simulink model "Copy_of_two_phase_main_loop"  (R2025b)
settings: Solver=VariableStepAuto  StartTime=0.0  StopTime=4000
undefined symbols (not defined in the file): cfg, u_cmd
libraries: nesl_utility x21, fl_lib x20, SimscapeFluids_lib x7, slpidlib x1
settings Model: LastModifiedBy=altoa
settings OptimizationCC: ZeroExternalMemoryAtStartup=off  ZeroInternalMemoryAtStartup=off
settings RTWCC: GenerateReport=on  LaunchReport=on  TargetLang=C++  CheckMdlBeforeBuild=Error
settings GRTTargetCC: TargetLangStandard=C++11 (ISO)  CodeInterfacePackaging=C++ class  SubcomponentCodeInterfacePackaging=C++ class

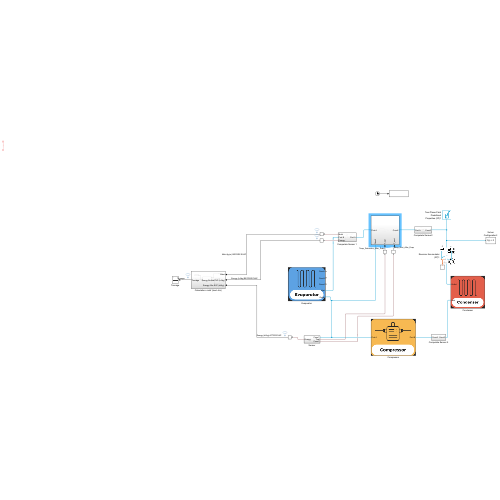
[thumbnail: Simulink's stored preview of the top-level diagram]
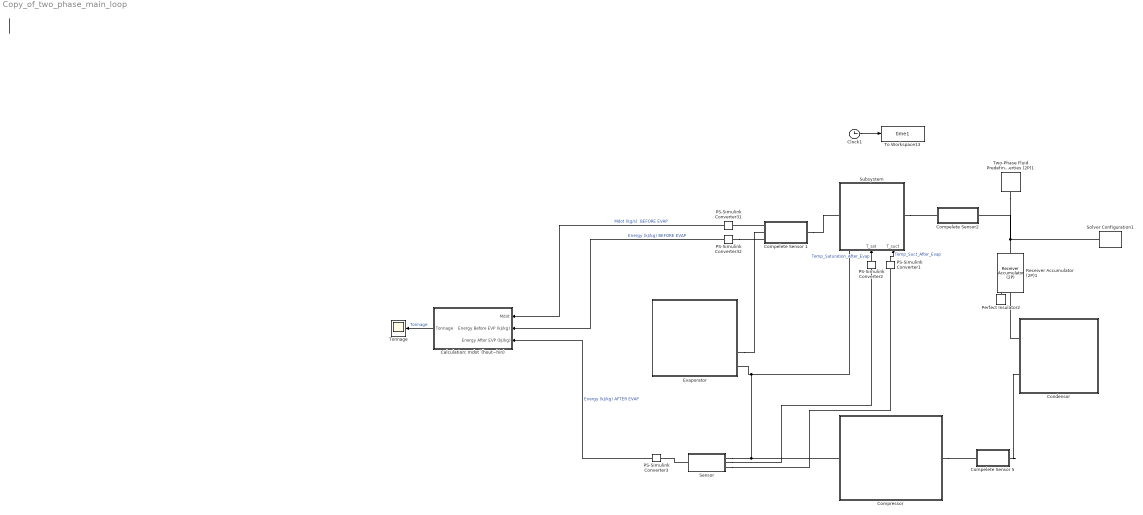
== system Copy_of_two_phase_main_loop ==
  Calculation: mdot˙(hout​−hin​) : Subsystem
  Clock1 : Clock
  Compelete Sensor 1 : Subsystem
  Compelete Sensor 5 : Subsystem
  Compelete Sensor2 : Subsystem
  Compressor : Subsystem
      mask Display: image('models\Icon\Compressor.png');
  Condensor : Subsystem
      mask Display: image('models\Icon\Condenser.png');
  Evaporator : Subsystem
      mask Display: image("models\Icon\Evaporator.png");
  PS-Simulink Converter{1..3,31..32} (5 alike) : nesl_utility/PS-Simulink Converter  PhysicalDomain=network_engine_domain  SubClassName=ps_output  LeftPortType=input  RightPortType=output  PseudoPeriodic=off  Frequencies=[]  VectorFormat=inherit  Unit=inherit  AffineConversion=off
  Perfect Insulator2 : fl_lib/Thermal/Thermal Elements/Perfect Insulator  T_specify=off  T_priority=None  T=293.15 K  T_nominal_specify=off  T_nominal_value=1  T_nominal_unit=K
  Receiver Accumulator (2P)1 : SimscapeFluids_lib/Two-Phase Fluid/Tanks & Accumulators/Receiver Accumulator (2P)  volume=pi*0.15^2/4 * 0.5 m^3  tank_area=pi*0.15^2/4 m^2  area_AV=pi*0.02^2/4 m^2  area_BV=pi*0.02^2/4 m^2  area_AL=pi*0.02^2/4 m^2  area_BL=pi*0.02^2/4 m^2  V_frac_liq_error=simscape.enum.assert.action.none  V_frac_liq_min=0.05  V_frac_liq_max=0.95  V_frac_smooth=0.05  p_crit_error=simscape.enum.assert.action.error  hc_vap=20 W/(K*m^2)  hc_liq=100 W/(K*m^2)  p_init=2.734 MPa  fraction_spec=fluids.two_phase_fluid.tanks_accumulators.enum.LiquidFractionSpec.Volume  M_frac_liq_init=0.5  V_frac_liq_init=0.5  saturated_init=true  energy_spec=fluids.two_phase_fluid.tanks_accumulators.enum.EnergySpec.SubcoolingSuperheating  delta_T_sub_init=5 deltaK  delta_T_sup_init=5 deltaK  T_liq_init=368.15 K  T_vap_init=378.15 K  h_liq_init=400 kJ/kg  h_vap_init=2700 kJ/kg  u_liq_init=400 kJ/kg  u_vap_init=2700 kJ/kg  tau_vap_cond=1 s
      settings: InternalSimscapePortConfiguration="{\"Bottom\":[],\"Left\":[{\"id\":\"AV\",\"label\":\"AV\",\"type\":\"foundation.two_phase_fluid.two_phase_fluid\"},{\"id\":\"AL\",\"label\":\"AL\",\"type\":\"foundation.two_phase_fluid.two_phase_fluid\"},{\"id\":\"H\",\"label\":\"H\",\"type\":\"foundation.thermal.thermal\"}],\"Right\":[{\"id\":\"BV\",\"label\":\"BV\",\"type\":\"foundation.two_phase_fluid.two_phase_fluid\"},{\"id\":\"BL\",\"label\":\"BL\",\"type\":\"foundation.two_phase_fluid.two_phase_fluid\"},{\"id\":\"L\",\"label\":\"L\",\"type\":\"output\"}],\"Top\":[]}"
  Sensor : Subsystem
  Solver Configuration1 : nesl_utility/Solver Configuration  PhysicalDomain=network_engine_domain  SubClassName=solver  LeftPortType=input  RightPortType=generic  Tones=[]  Harmonics=[]  SimulateNoise=off  Profile=off  UseLocalSampling=off  EnableSwitchedLinearOptims=on  FrequencyDomain=off  UseCCode=off  RelTol=0.001  AbsTol=0.001  MinStep=1e-09  ToWorkspace=off  RevertToSquareIcSolve=off  NumHomotopyIterations=100  PhasorMode=off  PhasorModeNumHarmonics=1  ConsistencySolver=NEWTON_FTOL  IndexReductionMethod=DerivativeReplacement  DoDC=off  ResidualTolerance=1e-09  ConsistencyTolSource=GLOBAL  ConsistencyAbsTol=0.001  ConsistencyRelTol=0.001  ConsistencyTolFactor=0.001  UseLocalSolver=off  LocalSolverChoice=NE_BACKWARD_EULER_ADVANCER  ResolveIndetEquations=on  FunctionEvalNumThread=1  LocalSolverSampleTime=0.001  DoFixedCost=off  MaxNonlinIter=3  MaxModeIter=2  ComputeImpulses=off  ImpulseIterations=2  LinearAlgebra=auto  LinearAlgebraNumThread=0  EquationFormulation=NE_TIME_EF  DelaysMemoryBudget=1024  AutomaticFiltering=on  FilteringTimeConstant=0.001  PartitionStorageMethod=AS_NEEDED  PartitionMemoryBudget=1024  PartitionMethod=ROBUST  MultibodyUseLocalSolver=off  MultibodyLocalSolverChoice=ODE1  MultibodyLocalSolverSampleTime=0.001
  Subsystem : Subsystem
      settings: PortSchema="{\"entries\":[{\"content\":{\"sides\":[{\"content\":{\"connectorIds\":[\"LConn1\"]},\"type\":\"ConnectorPlacement.EquallySpacedRectSide\",\"uuid\":\"f5d6d53e-9d0c-4e0a-9987-2cecb9078f40\"},{\"content\":{\"connectorIds\":[\"RConn1\"],\"side\":\"RIGHT\"},\"type\":\"ConnectorPlacement.EquallySpacedRectSide\",\"uuid\":\"a442d892-4933-408d-9a01-d57d967d5942\"},{\"content\":{\"side\":\"TOP\"},\"type\":\"ConnectorPlacement.EquallySpacedRectSide\",\"uuid\":\"9d728b22-2b02-46e5-9d77-02223002d615\"},{\"content\":{\"connectorIds\":[\"In1\",\"In2\",\"RConn2\"],\"side\":\"BOTTOM\"},\"type\":\"ConnectorPlacement.EquallySpacedRectSide\",\"uuid\":\"bdbf34ec-8662-4590-a2f3-7ce9740bfea5\"}]},\"type\":\"ConnectorPlacement.EquallySpacedConnector\",\"uuid\":\"3394dac1-307d-4ba8-b50d-5218a2108d88\"}],\"packageUris\":[\"http://schema.mathworks.com/mf0/Connector/R2020b\"],\"version\":\"1.0\"}"
  To Workspace13 : ToWorkspace  VariableName=time1  SampleTime=-1
  Tonnage : Scope
      settings: ActiveDisplayYMinimum=2.6000959343820402  ActiveDisplayYMaximum=3.4572001399689993  DataLoggingVariableName=ScopeData29
  Two-Phase Fluid Predefined Properties (2P)1 : SimscapeFluids_lib/Two-Phase Fluid/Utilities/Two-Phase Fluid Predefined Properties (2P)  fluid=fluids.two_phase_fluid.utilities.enum.Fluid.R32  p_atm=0.101325 MPa  properties_range_check=simscape.enum.assert.action.error  q_rev=0.01 Pa
  wires:
  Clock1/1 -> To Workspace13/1
  PS-Simulink Converter32/1 -> Calculation: mdot˙(hout​−hin​)/2(Energy Before EVP (kJ/kg))  "Energy (kJ/kg) BEFORE EVAP"
  Calculation: mdot˙(hout​−hin​)/1(Tonnage) -> Tonnage/1  "Tonnage"
  PS-Simulink Converter31/1 -> Calculation: mdot˙(hout​−hin​)/1(Mdot)  "Mdot (kg/s)  BEFORE EVAP"
  PS-Simulink Converter3/1 -> Calculation: mdot˙(hout​−hin​)/3("Energy After EVP (kJ/kg) ")  "Energy (kJ/kg) AFTER EVAP"
  PS-Simulink Converter1/1 -> Subsystem/1(T_suct)  "Temp_Suct_After_Evap"
  PS-Simulink Converter2/1 -> Subsystem/2(T_sat)  "Temp_Saturation_After_Evap"
  connections:
  ?
  Receiver Accumulator (2P)1/RConn2 -- Two-Phase Fluid Predefined Properties (2P)1/RConn1 -- Compelete Sensor2/LConn1 -- Solver Configuration1/RConn1
  Compelete Sensor 5/RConn1 -- Condensor/LConn2
  Perfect Insulator2/LConn1 -- Receiver Accumulator (2P)1/LConn3
  Compelete Sensor 1/RConn1 -- PS-Simulink Converter31/LConn1
  Evaporator/LConn4 -- Compelete Sensor 1/RConn2
  PS-Simulink Converter32/LConn1 -- Compelete Sensor 1/RConn3
  Condensor/LConn1 -- Receiver Accumulator (2P)1/LConn2
  Compressor/RConn1 -- Compelete Sensor 5/LConn1
  Sensor/RConn1 -- PS-Simulink Converter3/LConn1
  Sensor/LConn2 -- PS-Simulink Converter2/LConn1
  Sensor/LConn3 -- PS-Simulink Converter1/LConn1
  Sensor/LConn1 -- Evaporator/LConn5 -- Subsystem/RConn2 -- Compressor/LConn1
  Compelete Sensor 1/LConn1 -- Subsystem/RConn1
  Subsystem/LConn1 -- Compelete Sensor2/RConn1

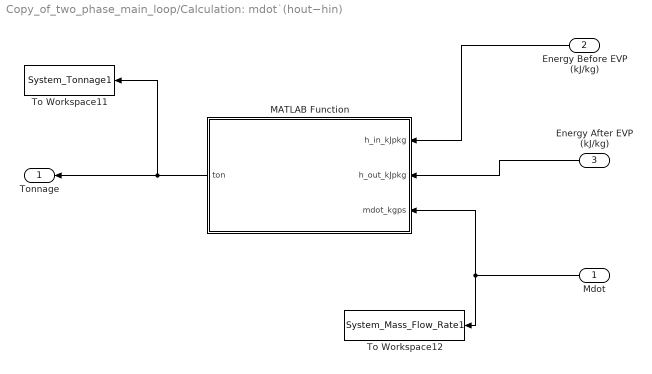
== system Copy_of_two_phase_main_loop/Calculation: mdot˙(hout​−hin​) ==
  Mdot : Inport
  Energy Before EVP (kJ/kg) : Inport  Port=2
  "Energy After EVP (kJ/kg) " : Inport  Port=3
  MATLAB Function : MATLAB Function  TreatAsAtomicUnit=on
  To Workspace11 : ToWorkspace  VariableName=System_Tonnage1  SampleTime=-1
  To Workspace12 : ToWorkspace  VariableName=System_Mass_Flow_Rate1  SampleTime=-1
  Tonnage : Outport
  wires:
  MATLAB Function/1(ton) -> To Workspace11/1, Tonnage/1
  Mdot/1 -> To Workspace12/1, MATLAB Function/3(mdot_kgps)
  Energy Before EVP (kJ/kg)/1 -> MATLAB Function/1(h_in_kJpkg)
  "Energy After EVP (kJ/kg) "/1 -> MATLAB Function/2(h_out_kJpkg)

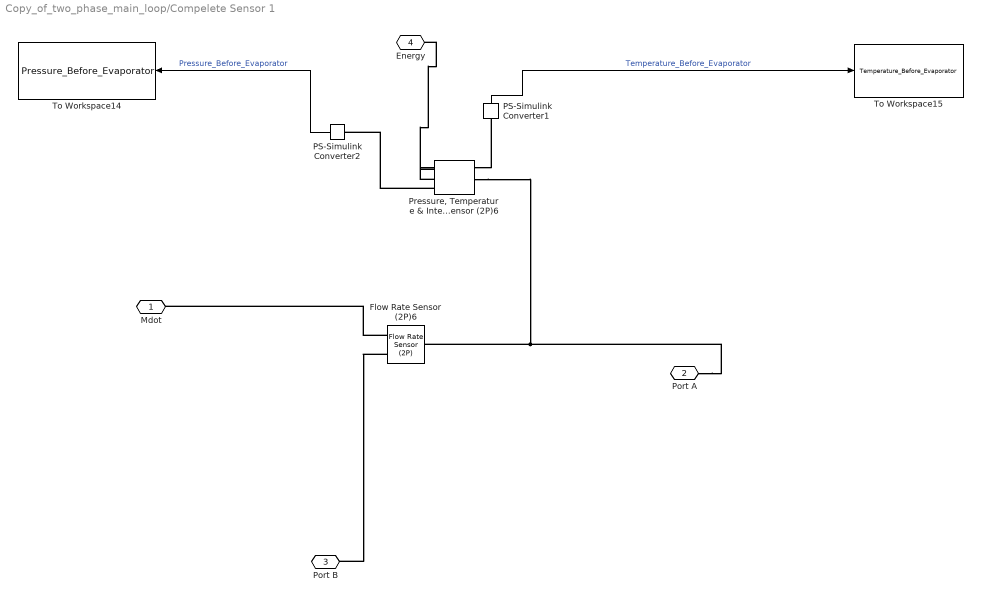
== system Copy_of_two_phase_main_loop/Compelete Sensor 1 ==
  Flow Rate Sensor (2P)6 : fl_lib/Two-Phase Fluid/Sensors/Flow Rate Sensor (2P)  mass_flow_measure=true  volumetric_flow_measure=false  energy_flow_measure=false
      settings: InternalSimscapePortConfiguration="{\"Bottom\":[],\"Left\":[{\"id\":\"A\",\"label\":\"A\",\"type\":\"foundation.two_phase_fluid.two_phase_fluid\"}],\"Right\":[{\"id\":\"B\",\"label\":\"B\",\"type\":\"foundation.two_phase_fluid.two_phase_fluid\"},{\"id\":\"M\",\"label\":\"M\",\"type\":\"output\"}],\"Top\":[]}"
  PS-Simulink Converter1 : nesl_utility/PS-Simulink Converter  PhysicalDomain=network_engine_domain  SubClassName=ps_output  LeftPortType=input  RightPortType=output  PseudoPeriodic=off  Frequencies=[]  VectorFormat=inherit  Unit=inherit  AffineConversion=off
  PS-Simulink Converter2 : nesl_utility/PS-Simulink Converter  PhysicalDomain=network_engine_domain  SubClassName=ps_output  LeftPortType=input  RightPortType=output  PseudoPeriodic=off  Frequencies=[]  VectorFormat=inherit  Unit=inherit  AffineConversion=off
  "Pressure, Temperature & Internal Energy Sensor (2P)6" : fl_lib/Two-Phase Fluid/Sensors/Pressure, Temperature & Internal Energy Sensor (2P)  reference=foundation.enum.MeasurementReference.absolute  pressure=true  pressure_spec=foundation.enum.PressureMeasementSpec.Absolute  temperature=true  internal_energy=true
      settings: InternalSimscapePortConfiguration="{\"Bottom\":[{\"id\":\"T\",\"label\":\"T\",\"type\":\"output\"},{\"id\":\"U\",\"label\":\"U\",\"type\":\"output\"}],\"Left\":[{\"id\":\"A\",\"label\":\"A\",\"type\":\"foundation.two_phase_fluid.two_phase_fluid\"}],\"Right\":[{\"id\":\"Pa\",\"label\":\"Pa\",\"type\":\"output\"}],\"Top\":[]}"
  To Workspace14 : ToWorkspace  VariableName=Pressure_Before_Evaporator  SampleTime=-1
  To Workspace15 : ToWorkspace  VariableName=Temperature_Before_Evaporator  SampleTime=-1
  Mdot : PMIOPort  Side=Right
  Port A : PMIOPort  Port=2  Side=Left
  Port B : PMIOPort  Port=3  Side=Right
  "Energy " : PMIOPort  Port=4  Side=Right
  wires:
  PS-Simulink Converter1/1 -> To Workspace15/1  "Temperature_Before_Evaporator"
  PS-Simulink Converter2/1 -> To Workspace14/1  "Pressure_Before_Evaporator"
  connections:
  Port A/RConn1 -- "Pressure, Temperature & Internal Energy Sensor (2P)6"/LConn1 -- Flow Rate Sensor (2P)6/LConn1
  Flow Rate Sensor (2P)6/RConn1 -- Port B/RConn1
  Flow Rate Sensor (2P)6/RConn2 -- Mdot/RConn1
  "Pressure, Temperature & Internal Energy Sensor (2P)6"/RConn3 -- "Energy "/RConn1
  "Pressure, Temperature & Internal Energy Sensor (2P)6"/RConn2 -- PS-Simulink Converter1/LConn1
  "Pressure, Temperature & Internal Energy Sensor (2P)6"/RConn1 -- PS-Simulink Converter2/LConn1

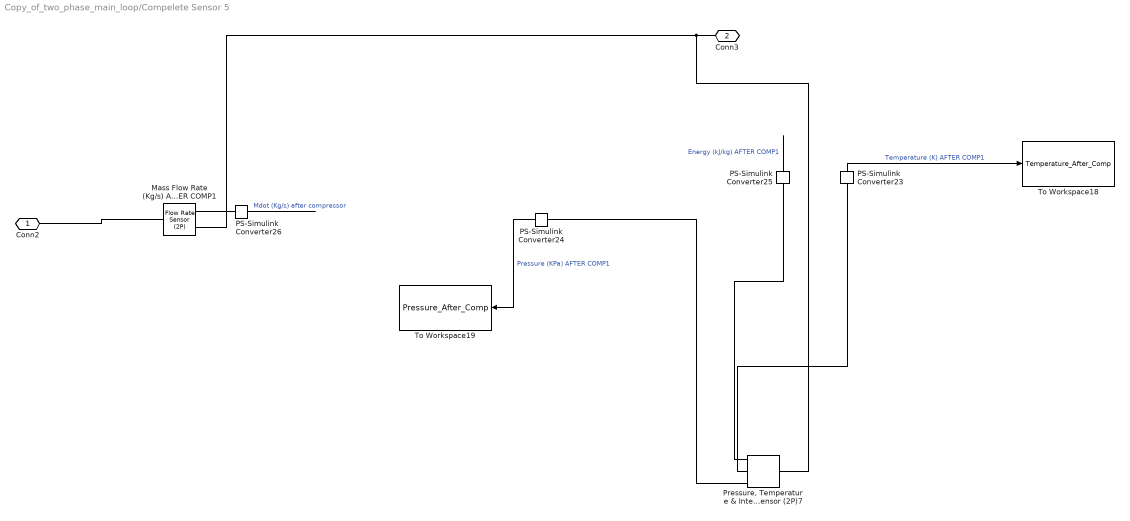
== system Copy_of_two_phase_main_loop/Compelete Sensor 5 ==
  Mass Flow Rate (Kg/s) AFTER COMP1 : fl_lib/Two-Phase Fluid/Sensors/Flow Rate Sensor (2P)  mass_flow_measure=true  volumetric_flow_measure=false  energy_flow_measure=false
      settings: InternalSimscapePortConfiguration="{\"Bottom\":[],\"Left\":[{\"id\":\"A\",\"label\":\"A\",\"type\":\"foundation.two_phase_fluid.two_phase_fluid\"}],\"Right\":[{\"id\":\"B\",\"label\":\"B\",\"type\":\"foundation.two_phase_fluid.two_phase_fluid\"},{\"id\":\"M\",\"label\":\"M\",\"type\":\"output\"}],\"Top\":[]}"
  PS-Simulink Converter{23..26} (4 alike) : nesl_utility/PS-Simulink Converter  PhysicalDomain=network_engine_domain  SubClassName=ps_output  LeftPortType=input  RightPortType=output  PseudoPeriodic=off  Frequencies=[]  VectorFormat=inherit  Unit=inherit  AffineConversion=off
  "Pressure, Temperature & Internal Energy Sensor (2P)7" : fl_lib/Two-Phase Fluid/Sensors/Pressure, Temperature & Internal Energy Sensor (2P)  reference=foundation.enum.MeasurementReference.absolute  pressure=true  pressure_spec=foundation.enum.PressureMeasementSpec.Absolute  temperature=true  internal_energy=true
      settings: InternalSimscapePortConfiguration="{\"Bottom\":[{\"id\":\"T\",\"label\":\"T\",\"type\":\"output\"},{\"id\":\"U\",\"label\":\"U\",\"type\":\"output\"}],\"Left\":[{\"id\":\"A\",\"label\":\"A\",\"type\":\"foundation.two_phase_fluid.two_phase_fluid\"}],\"Right\":[{\"id\":\"Pa\",\"label\":\"Pa\",\"type\":\"output\"}],\"Top\":[]}"
  To Workspace18 : ToWorkspace  VariableName=Temperature_After_Comp  SampleTime=-1
  To Workspace19 : ToWorkspace  VariableName=Pressure_After_Comp  SampleTime=-1
  Conn2 : PMIOPort  Side=Left
  Conn3 : PMIOPort  Port=2  Side=Right
  wires:
  PS-Simulink Converter26/1 -> ?  "Mdot (Kg/s) after compressor"
  PS-Simulink Converter24/1 -> To Workspace19/1  "Pressure (KPa) AFTER COMP1"
  PS-Simulink Converter23/1 -> To Workspace18/1  "Temperature (K) AFTER COMP1"
  PS-Simulink Converter25/1 -> ?  "Energy (kJ/kg) AFTER COMP1"
  connections:
  Conn2/RConn1 -- Mass Flow Rate (Kg/s) AFTER COMP1/LConn1
  PS-Simulink Converter26/LConn1 -- Mass Flow Rate (Kg/s) AFTER COMP1/RConn2
  Mass Flow Rate (Kg/s) AFTER COMP1/RConn1 -- Conn3/RConn1 -- "Pressure, Temperature & Internal Energy Sensor (2P)7"/LConn1
  PS-Simulink Converter23/LConn1 -- "Pressure, Temperature & Internal Energy Sensor (2P)7"/RConn2
  PS-Simulink Converter25/LConn1 -- "Pressure, Temperature & Internal Energy Sensor (2P)7"/RConn3
  PS-Simulink Converter24/LConn1 -- "Pressure, Temperature & Internal Energy Sensor (2P)7"/RConn1

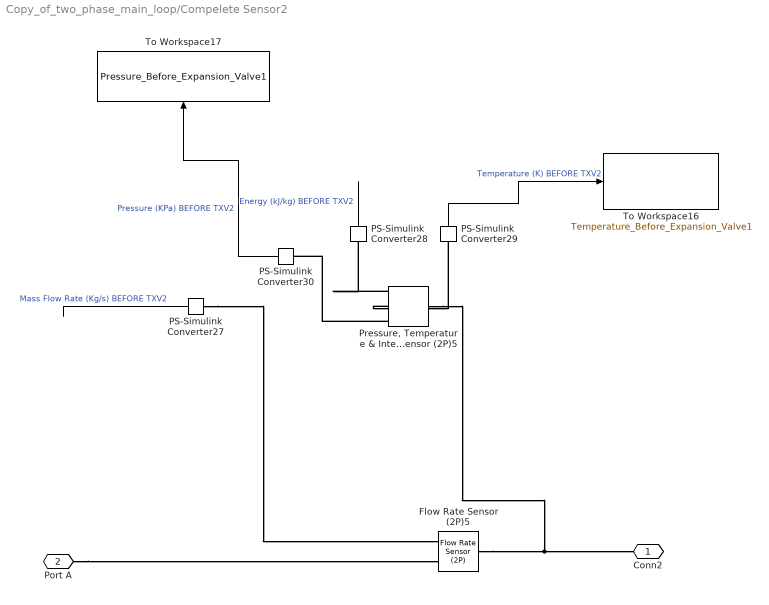
== system Copy_of_two_phase_main_loop/Compelete Sensor2 ==
  Flow Rate Sensor (2P)5 : fl_lib/Two-Phase Fluid/Sensors/Flow Rate Sensor (2P)  mass_flow_measure=true  volumetric_flow_measure=false  energy_flow_measure=false
      settings: InternalSimscapePortConfiguration="{\"Bottom\":[],\"Left\":[{\"id\":\"A\",\"label\":\"A\",\"type\":\"foundation.two_phase_fluid.two_phase_fluid\"}],\"Right\":[{\"id\":\"B\",\"label\":\"B\",\"type\":\"foundation.two_phase_fluid.two_phase_fluid\"},{\"id\":\"M\",\"label\":\"M\",\"type\":\"output\"}],\"Top\":[]}"
  PS-Simulink Converter{27..30} (4 alike) : nesl_utility/PS-Simulink Converter  PhysicalDomain=network_engine_domain  SubClassName=ps_output  LeftPortType=input  RightPortType=output  PseudoPeriodic=off  Frequencies=[]  VectorFormat=inherit  Unit=inherit  AffineConversion=off
  "Pressure, Temperature & Internal Energy Sensor (2P)5" : fl_lib/Two-Phase Fluid/Sensors/Pressure, Temperature & Internal Energy Sensor (2P)  reference=foundation.enum.MeasurementReference.absolute  pressure=true  pressure_spec=foundation.enum.PressureMeasementSpec.Absolute  temperature=true  internal_energy=true
      settings: InternalSimscapePortConfiguration="{\"Bottom\":[{\"id\":\"T\",\"label\":\"T\",\"type\":\"output\"},{\"id\":\"U\",\"label\":\"U\",\"type\":\"output\"}],\"Left\":[{\"id\":\"A\",\"label\":\"A\",\"type\":\"foundation.two_phase_fluid.two_phase_fluid\"}],\"Right\":[{\"id\":\"Pa\",\"label\":\"Pa\",\"type\":\"output\"}],\"Top\":[]}"
  To Workspace16 : ToWorkspace  VariableName=Temperature_Before_Expansion_Valve1  SampleTime=-1
  To Workspace17 : ToWorkspace  VariableName=Pressure_Before_Expansion_Valve1  SampleTime=-1
  Conn2 : PMIOPort  Side=Left
  Port A : PMIOPort  Port=2  Side=Right
  wires:
  PS-Simulink Converter30/1 -> To Workspace17/1  "Pressure (KPa) BEFORE TXV2"
  PS-Simulink Converter29/1 -> To Workspace16/1  "Temperature (K) BEFORE TXV2"
  PS-Simulink Converter27/1 -> ?  "Mass Flow Rate (Kg/s) BEFORE TXV2"
  PS-Simulink Converter28/1 -> ?  "Energy (kJ/kg) BEFORE TXV2"
  connections:
  Port A/RConn1 -- Flow Rate Sensor (2P)5/RConn1
  PS-Simulink Converter27/LConn1 -- Flow Rate Sensor (2P)5/RConn2
  Flow Rate Sensor (2P)5/LConn1 -- "Pressure, Temperature & Internal Energy Sensor (2P)5"/LConn1 -- Conn2/RConn1
  "Pressure, Temperature & Internal Energy Sensor (2P)5"/RConn1 -- PS-Simulink Converter30/LConn1
  "Pressure, Temperature & Internal Energy Sensor (2P)5"/RConn2 -- PS-Simulink Converter29/LConn1
  "Pressure, Temperature & Internal Energy Sensor (2P)5"/RConn3 -- PS-Simulink Converter28/LConn1

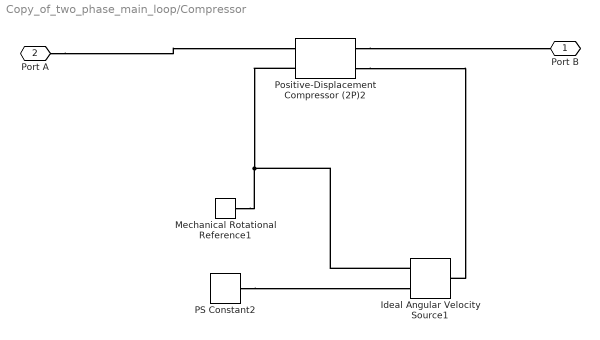
== system Copy_of_two_phase_main_loop/Compressor ==
  Ideal Angular Velocity Source1 : fl_lib/Mechanical/Mechanical Sources/Ideal Angular Velocity Source
  Mechanical Rotational Reference1 : fl_lib/Mechanical/Rotational Elements/Mechanical Rotational Reference
  PS Constant2 : fl_lib/Physical Signals/Sources/PS Constant  constant=220 Hz
  Positive-Displacement Compressor (2P)2 : SimscapeFluids_lib/Two-Phase Fluid/Fluid Machines/Positive-Displacement Compressor (2P)  dispSpec=fluids.two_phase_fluid.fluid_machines.enum.DisplacementSpecification.FlowSpeed  v_disp=130 cm^3/rev  mdot_nom=0.013 kg/s  omega_nom=60 Hz  efficiencySpec=fluids.two_phase_fluid.fluid_machines.enum.VolumetricEfficiencyParameterization.Analytical  thermodynamicModelSpec=fluids.two_phase_fluid.fluid_machines.enum.ThermodynamicModel.Polytropic  n=1.2  eta_isen=0.65  eta_isen_TLU=[.95, .9, .85, .8, .75; .925, .875, .825, .775, .725; .875, .825, .775, .725, .675; .75, .7, .65, .6, .55]  eta_vol_nom=0.9  pr_TLU=[2, 4, 6, 8]  omega_TLU=[800, 1500, 2800, 3300, 4000] rpm  eta_vol_TLU=[.95, .9, .85, .8, .75; .925, .875, .825, .775, .725; .875, .825, .775, .725, .675; .75, .7, .65, .6, .55]  nominalSpec=fluids.two_phase_fluid.fluid_machines.enum.NominalConditionsSpecification.SaturationTemperatures  pr_nom=5  p_in_nom=0.101325 MPa  T_in_nom=373.15 K  T_evap_nom=5 degC  T_cond_nom=45 degC  delta_T_nom=5 deltaK  mechanical_efficiency=0.9  area_A=pi*0.02^2/4 m^2  area_B=pi*0.02^2/4 m^2  VaporCheck=simscape.enum.assert.action.warn
      settings: InternalSimscapePortConfiguration="{\"Bottom\":[],\"Left\":[{\"id\":\"A\",\"label\":\"A\",\"type\":\"foundation.two_phase_fluid.two_phase_fluid\"},{\"id\":\"C\",\"label\":\"C\",\"type\":\"foundation.mechanical.rotational.rotational\"}],\"Right\":[{\"id\":\"B\",\"label\":\"B\",\"type\":\"foundation.two_phase_fluid.two_phase_fluid\"},{\"id\":\"R\",\"label\":\"R\",\"type\":\"foundation.mechanical.rotational.rotational\"}],\"Top\":[]}"
  Port B : PMIOPort  Side=Right
  Port A : PMIOPort  Port=2  Side=Left
  connections:
  Positive-Displacement Compressor (2P)2/RConn1 -- Port B/RConn1
  Port A/RConn1 -- Positive-Displacement Compressor (2P)2/LConn1
  Ideal Angular Velocity Source1/RConn2 -- Mechanical Rotational Reference1/LConn1 -- Positive-Displacement Compressor (2P)2/LConn2
  Positive-Displacement Compressor (2P)2/RConn2 -- Ideal Angular Velocity Source1/LConn1
  PS Constant2/RConn1 -- Ideal Angular Velocity Source1/RConn1

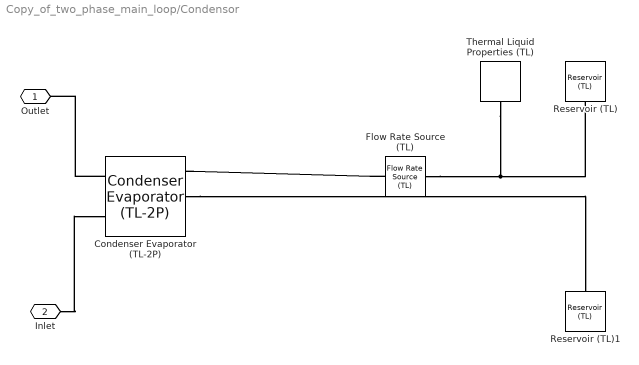
== system Copy_of_two_phase_main_loop/Condensor ==
  Condenser Evaporator (TL-2P) : SimscapeFluids_lib/Heat Exchangers/Two-Phase Fluid - Thermal Liquid/Condenser Evaporator (TL-2P)  flow_arrangement=fluids.heat_exchangers.enum.FlowArrangementTL2P.Counter  cross_flow_arrangement=fluids.heat_exchangers.enum.CrossFlowArrangementTL2P.UnmixedUnmixed  R_wall=0 K/kW  wall_thermal_mass=true  mass_wall=92.658 kg  cp_wall="385      J/(K*kg)"  area_A1=13 * (pi *0.01^2 / 4); m^2  area_B1=13 * (pi *0.01^2 / 4); m^2  area_A2=0.0011 m^2  area_B2=0.0011 m^2  flow_geometry_TL=fluids.heat_exchangers.enum.FlowGeometryTL.InsideTubes  tube_num_TL=13  tube_length_TL=9.5 m  tube_cross_section_TL=fluids.heat_exchangers.enum.TubeCrossSection.Circular  tube_diameter_TL=0.0100 m  tube_width_TL=0.05 m  tube_height_TL=0.05 m  tube_inner_diameter_TL=0.05 m  tube_outer_diameter_TL=0.1 m  tube_flow_area_TL=0.002 m^2  tube_wetted_perimeter_TL=0.15 m  tube_heat_perimeter_TL=0.15 m  tube_pressure_loss_spec_TL=fluids.heat_exchangers.enum.TubePressureLossSpec.Haaland  tube_loss_coeff_TL=10  tube_local_pressure_loss_spec_TL=fluids.heat_exchangers.enum.LocalLossSpec.AggregateLength  tube_length_add_TL=0.1 m  tube_local_loss_coefficient_TL=0.1  tube_roughness_pressure_TL=15e-6 m  tube_Re_lam_pressure_TL=2000  tube_Re_tur_pressure_TL=4000  tube_shape_factor_generic_TL=64  tube_heat_coeff_spec_TL=fluids.heat_exchangers.enum.TubeHeatCoeffSpec.Gneilinski  tube_colburn_coeff_TL=[.023, .8, .33]  tube_roughness_heat_TL=15e-6 m  tube_Re_lam_heat_TL=2000  tube_Re_tur_heat_TL=4000  tube_Nu_lam_generic_TL=3.66  bank_arrangement_TL=fluids.heat_exchangers.enum.BankArrangement.Inline  bank_num_rows_TL=5  bank_tubes_per_row_TL=5  bank_width_TL=1 m  bank_tube_diameter_TL=0.05 m  bank_longitudinal_pitch_TL=0.15 m  bank_transverse_pitch_TL=0.15 m  bank_pressure_loss_spec_TL=fluids.heat_exchangers.enum.BankPressureLossSpec.Martin  bank_euler_TL=10  bank_heat_coeff_spec_TL=fluids.heat_exchangers.enum.BankHeatCoeffSpec.Martin  bank_colburn_coeff_TL=[.27, .63, .36]  generic_flow_area_TL=0.01 m^2  generic_heat_area_TL=2 m^2  generic_volume_TL=0.05 m^3  generic_loss_coeff_TL=10  generic_colburn_coeff_TL=[.023, .8, .33]  fouling_factor_TL=0 K*m^2/kW  fin_area_TL=0 m^2  fin_efficiency_TL=0.5  p_init_TL=2e5 Pa  T_init_TL=303.15 K  tube_num_2P=22  tube_length_2P=9.5 m  tube_cross_section_2P=fluids.heat_exchangers.enum.TubeCrossSection.Circular  tube_diameter_2P=0.008 m  tube_width_2P=0.05 m  tube_height_2P=0.05 m  tube_inner_diameter_2P=0.05 m  tube_outer_diameter_2P=0.1 m  tube_flow_area_2P=0.002 m^2  tube_wetted_perimeter_2P=0.15 m  tube_heat_perimeter_2P=0.15 m  tube_pressure_loss_spec_2P=fluids.heat_exchangers.enum.TubePressureLossSpec2P.Haaland  tube_loss_coeff_2P=10  tube_local_pressure_loss_spec_2P=fluids.heat_exchangers.enum.LocalLossSpec.AggregateLength  tube_length_add_2P=0.1 m  tube_local_loss_coefficient_2P=0.1  tube_roughness_pressure_2P=15e-6 m  tube_Re_lam_pressure_2P=2000  tube_Re_tur_pressure_2P=4000  tube_shape_factor_generic_2P=64  tube_heat_coeff_spec_2P=fluids.heat_exchangers.enum.TubeHeatCoeffSpec2P.GneilinskiCavalliniZecchin  tube_colburn_coeff_liq_2P=[.023, .8, .33]  tube_colburn_coeff_mix_2P=[.05, .8, .33]  tube_colburn_coeff_vap_2P=[.023, .8, .33]  tube_roughness_heat_2P=15e-6 m  tube_Re_lam_heat_2P=2000  tube_Re_tur_heat_2P=4000  tube_Nu_lam_generic_2P=3.66  fouling_factor_2P=0 K*m^2/kW  fin_area_2P=0 m^2  fin_efficiency_2P=0.5  energy_spec_2P=foundation.enum.energy_spec.temperature  p_init_2P=2.5e6 Pa  T_init_2P=293.15 K  x_init_2P=0.5  alpha_init_2P=0.5  h_init_2P=1500 kJ/kg  u_init_2P=1500 kJ/kg
      settings: InternalSimscapePortConfiguration="{\"Bottom\":[],\"Left\":[{\"id\":\"A1\",\"label\":\"A1\",\"type\":\"foundation.thermal_liquid.thermal_liquid\"},{\"id\":\"B1\",\"label\":\"B1\",\"type\":\"foundation.thermal_liquid.thermal_liquid\"}],\"Right\":[{\"id\":\"A2\",\"label\":\"A2\",\"type\":\"foundation.two_phase_fluid.two_phase_fluid\"},{\"id\":\"B2\",\"label\":\"B2\",\"type\":\"foundation.two_phase_fluid.two_phase_fluid\"}],\"Top\":[{\"id\":\"Z\",\"label\":\"Z\",\"type\":\"output\"}]}"
  Flow Rate Source (TL) : fl_lib/Thermal Liquid/Sources/Flow Rate Source (TL)  source_type=foundation.enum.constant_controlled.constant  flow_type=foundation.enum.mass_volumetric_flow.mass  mass_flow=0.8 kg/s  volumetric_flow=0 m^3/s  power_spec=foundation.enum.power_spec.isentropic  area=0.0011 m^2
      settings: InternalSimscapePortConfiguration="{\"Bottom\":[],\"Left\":[{\"id\":\"A\",\"label\":\"A\",\"type\":\"foundation.thermal_liquid.thermal_liquid\"}],\"Right\":[{\"id\":\"B\",\"label\":\"B\",\"type\":\"foundation.thermal_liquid.thermal_liquid\"}],\"Top\":[]}"
  Reservoir (TL) : fl_lib/Thermal Liquid/Elements/Reservoir (TL)  pressure_spec=foundation.enum.pressure_spec.specified  reservoir_pressure=2e5 Pa  reservoir_temperature=30 degC  area=0.0011 m^2
  Reservoir (TL)1 : fl_lib/Thermal Liquid/Elements/Reservoir (TL)  pressure_spec=foundation.enum.pressure_spec.specified  reservoir_pressure=2e5 Pa  reservoir_temperature=35 degC  area=0.0011 m^2
  Thermal Liquid Properties (TL) : SimscapeFluids_lib/Thermal Liquid/Utilities/Thermal Liquid Properties (TL)  fluid_list=fluids.thermal_liquid.utilities.enum.thermal_liquid_fluid_list.water  concentration_param_EG=fluids.thermal_liquid.utilities.enum.thermal_liquid_concentration.volume_fraction  concentration_param_PG=fluids.thermal_liquid.utilities.enum.thermal_liquid_concentration.volume_fraction  c_mass_SW=3.5e-3  c_mass_EG=0.1  c_mass_PG=0.1  c_mass_GL=0.1  c_vol_EG=0.1  c_vol_PG=0.1  beta_const_EG=2.1791 GPa  beta_const_PG=2.1791 GPa  beta_const_GL=2.1791 GPa  p_min_EG=0.01 MPa  p_min_PG=0.01 MPa  p_min_GL=0.01 MPa  p_max_EG=50 MPa  p_max_PG=50 MPa  p_max_GL=50 MPa  p_atm=0.101325 MPa  properties_range_check=simscape.enum.assert.action.error
  Outlet : PMIOPort  Side=Left
  Inlet : PMIOPort  Port=2  Side=Left
  connections:
  Inlet/RConn1 -- Condenser Evaporator (TL-2P)/RConn2
  Condenser Evaporator (TL-2P)/RConn1 -- Outlet/RConn1
  Thermal Liquid Properties (TL)/RConn1 -- Flow Rate Source (TL)/LConn1 -- Reservoir (TL)/LConn1
  Condenser Evaporator (TL-2P)/LConn2 -- Reservoir (TL)1/LConn1
  Flow Rate Source (TL)/RConn1 -- Condenser Evaporator (TL-2P)/LConn1

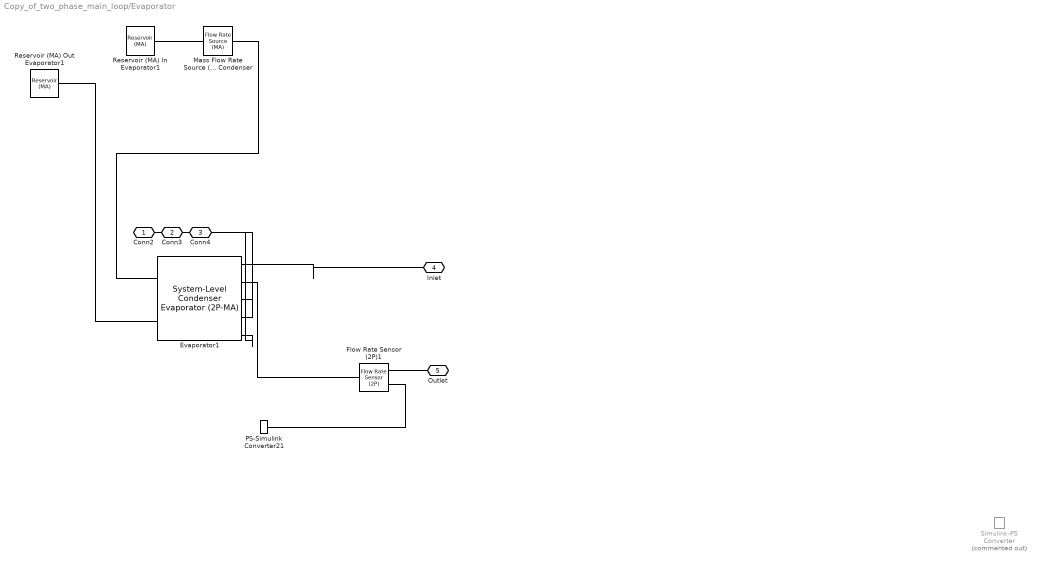
== system Copy_of_two_phase_main_loop/Evaporator ==
  Evaporator1 : SimscapeFluids_lib/Heat Exchangers/Two-Phase Fluid - Moist Air/System-Level Condenser Evaporator (2P-MA)  flow_arrangement=fluids.heat_exchangers.enum.SystemLevelFlowArrangement2PMA.Cross  wall_thermal_mass=simscape.enum.onoff.off  mass_wall=1 kg  cp_wall=490 J/(K*kg)  nominal_init_wall=true  T_wall_init=293.15 K  area_A1=pi*0.02^2/4 m^2  area_B1=pi*0.02^2/4 m^2  area_A2=0.4^2 m^2  area_B2=0.4^2 m^2  operating_condition_2P=fluids.heat_exchangers.enum.SystemLevelOperatingCondition2PMA.Evaporator  mdot_nominal_2P=0.04 kg/s  delta_p_nominal_2P=0.01 MPa  pressure_spec_cond_2P=fluids.heat_exchangers.enum.SystemLevelPressureSpecCondenser2P.InletPressure  pressure_spec_evap_2P=fluids.heat_exchangers.enum.SystemLevelPressureSpecEvaporator2P.EvaporatingTemperature  p_in_nominal_2P=1 MPa  T_cond_nominal_2P=313.15 K  T_evap_nominal_2P=10 degC  inlet_spec_2P=fluids.heat_exchangers.enum.SystemLevelInletSpec2P.Enthalpy  T_in_nominal_2P=333.15 K  h_in_nominal_2P=267 kJ/kg  x_in_nominal_2P=1  capacity_spec_2P=fluids.heat_exchangers.enum.SystemLevelCapacitySpec.OutletCondition  Q_nominal=0.1 kW  outlet_spec_cond_2P=fluids.heat_exchangers.enum.SystemLevelOutletSpecCondenser2P.Enthalpy  outlet_spec_evap_2P=fluids.heat_exchangers.enum.SystemLevelOutletSpecEvaporator2P.Superheating  delta_T_sub_nominal_2P=5 deltaK  delta_T_sup_nominal_2P=5 deltaK  h_out_nominal_2P=250 kJ/kg  x_out_nominal_2P=0  volume_2P=0.001 m^3  nominal_init_2P=true  energy_spec_2P=foundation.enum.energy_spec.enthalpy  p_init_2P=0.101325 MPa  T_init_2P=293.15 K  x_init_2P=0.5  alpha_init_2P=0.5  h_init_2P=1500 kJ/kg  u_init_2P=1500 kJ/kg  mdot_nominal_MA=1.2 * 1.2 kg/s  delta_p_nominal_MA=0.001 MPa  p_in_nominal_MA=0.101325 MPa  T_in_nominal_MA=22 degC  inlet_humidity_spec_MA=foundation.enum.HumiditySpec.RelativeHumidity  RH_in_nominal_MA=0.5  x_w_in_nominal_MA=0.01  y_w_in_nominal_MA=0.01  HR_in_nominal_MA=0.01  Tw_in_nominal_MA=287 K  inlet_trace_gas_spec_MA=foundation.enum.trace_gas_spec.mole_fraction  x_g_in_nominal_MA=0.001  y_g_in_nominal_MA=0  volume_MA=0.1 m^3  nominal_init_MA=true  p_init_MA=0.101325 MPa  T_init_MA=293.15 K  humidity_spec_MA=foundation.enum.HumiditySpec.RelativeHumidity  RH_init_MA=0.5  x_w_init_MA=0.01  y_w_init_MA=0.01  HR_init_MA=0.01  Tw_init_MA=287 K  trace_gas_spec_MA=foundation.enum.trace_gas_spec.mass_fraction  x_g_init_MA=0.001  y_g_init_MA=0.001  r_d_init_MA=0  RH_ws_MA=1  time_constant_cond_MA=1e-3 s  time_constant_evap_MA=1e-3 s  fraction_entrained_MA=1  a_liq_2P=0.023  a_mix_2P=0.005  a_vap_2P=0.023  b_2P=0.8  c_2P=0.33  a_MA=0.023  b_MA=0.8  c_MA=0.33
      settings: InternalSimscapePortConfiguration="{\"Bottom\":[],\"Left\":[{\"id\":\"A1\",\"label\":\"A1\",\"type\":\"foundation.two_phase_fluid.two_phase_fluid\"},{\"id\":\"B1\",\"label\":\"B1\",\"type\":\"foundation.two_phase_fluid.two_phase_fluid\"}],\"Right\":[{\"id\":\"A2\",\"label\":\"A2\",\"type\":\"foundation.moist_air.moist_air\"},{\"id\":\"B2\",\"label\":\"B2\",\"type\":\"foundation.moist_air.moist_air\"}],\"Top\":[{\"id\":\"Q1\",\"label\":\"Q1\",\"type\":\"output\"},{\"id\":\"Q2\",\"label\":\"Q2\",\"type\":\"output\"},{\"id\":\"W\",\"label\":\"W\",\"type\":\"output\"}]}"
  Flow Rate Sensor (2P)1 : fl_lib/Two-Phase Fluid/Sensors/Flow Rate Sensor (2P)  mass_flow_measure=true  volumetric_flow_measure=false  energy_flow_measure=false
      settings: InternalSimscapePortConfiguration="{\"Bottom\":[],\"Left\":[{\"id\":\"A\",\"label\":\"A\",\"type\":\"foundation.two_phase_fluid.two_phase_fluid\"}],\"Right\":[{\"id\":\"B\",\"label\":\"B\",\"type\":\"foundation.two_phase_fluid.two_phase_fluid\"},{\"id\":\"M\",\"label\":\"M\",\"type\":\"output\"}],\"Top\":[]}"
  Mass Flow Rate Source (MA) Condenser : fl_lib/Moist Air/Sources/Flow Rate Source (MA)  source_type=foundation.enum.constant_controlled.constant  flow_type=foundation.enum.mass_volumetric_flow.mass  mass_flow=1.2 * 1.5 kg/s  volumetric_flow=0 m^3/s  volumetric_flow_conditions=foundation.enum.volumetric_flow_conditions.actual  p_std=0.101325 MPa  T_std=20 degC  RH_std=0.65  power_spec=foundation.enum.power_spec.none  area_A=0.4^2 m^2  area_B=0.4^2 m^2
      settings: InternalSimscapePortConfiguration="{\"Bottom\":[],\"Left\":[{\"id\":\"A\",\"label\":\"A\",\"type\":\"foundation.moist_air.moist_air\"}],\"Right\":[{\"id\":\"B\",\"label\":\"B\",\"type\":\"foundation.moist_air.moist_air\"}],\"Top\":[]}"
  PS-Simulink Converter21 : nesl_utility/PS-Simulink Converter  PhysicalDomain=network_engine_domain  SubClassName=ps_output  LeftPortType=input  RightPortType=output  PseudoPeriodic=off  Frequencies=[]  VectorFormat=inherit  Unit=inherit  AffineConversion=off
  Reservoir (MA) In Evaporator1 : fl_lib/Moist Air/Elements/Reservoir (MA)  pressure_input=false  pressure_spec=foundation.enum.pressure_spec.atmospheric  reservoir_pressure=0.101325 MPa  temperature_input=false  temperature_spec=foundation.enum.temperature_spec.specified  reservoir_temperature=22 degC  humidity_input=false  humidity_spec=foundation.enum.HumiditySpec.RelativeHumidity  reservoir_RH=0.5  reservoir_x_w=0.01  reservoir_y_w=0.01  reservoir_HR=0.01  reservoir_Tw=287 K  trace_gas_input=false  trace_gas_spec=foundation.enum.trace_gas_spec.mole_fraction  reservoir_x_g=0.001  reservoir_y_g=0  water_droplets_input=false  reservoir_r_d=0  RH_ws=1  area_A=0.4^2 m^2  input_error_spec=foundation.enum.input_range_error.warn
  Reservoir (MA) Out Evaporator1 : fl_lib/Moist Air/Elements/Reservoir (MA)  pressure_input=false  pressure_spec=foundation.enum.pressure_spec.atmospheric  reservoir_pressure=0.101325 MPa  temperature_input=false  temperature_spec=foundation.enum.temperature_spec.specified  reservoir_temperature=20 degC  humidity_input=false  humidity_spec=foundation.enum.HumiditySpec.RelativeHumidity  reservoir_RH=0.5  reservoir_x_w=0.01  reservoir_y_w=0.01  reservoir_HR=0.01  reservoir_Tw=287 K  trace_gas_input=false  trace_gas_spec=foundation.enum.trace_gas_spec.mole_fraction  reservoir_x_g=0.001  reservoir_y_g=0  water_droplets_input=false  reservoir_r_d=0  RH_ws=1  area_A=0.4^2 m^2  input_error_spec=foundation.enum.input_range_error.warn
  Simulink-PS Converter : nesl_utility/Simulink-PS Converter  Commented=on  PhysicalDomain=network_engine_domain  SubClassName=ps_input  LeftPortType=input  RightPortType=output  PseudoPeriodic=off  Frequencies=[]  NoiseDistribution=none  NoiseParameters=[]  Unit=W/(K*m^2)  AffineConversion=off  FilteringAndDerivatives=provide  SimscapeFilterOrder=1  InputFilterTimeConstant=0.001  UdotUserProvided=0
  Conn2 : PMIOPort  Side=Left
  Conn3 : PMIOPort  Port=2  Side=Left
  Conn4 : PMIOPort  Port=3  Side=Left
  Inlet : PMIOPort  Port=4  Side=Left
  Outlet : PMIOPort  Port=5  Side=Left
  connections:
  Evaporator1/LConn3 -- Conn4/RConn1
  Evaporator1/LConn4 -- Conn3/RConn1
  Evaporator1/LConn5 -- Conn2/RConn1
  Reservoir (MA) Out Evaporator1/LConn1 -- Evaporator1/RConn2
  Reservoir (MA) In Evaporator1/LConn1 -- Mass Flow Rate Source (MA) Condenser/LConn1
  Mass Flow Rate Source (MA) Condenser/RConn1 -- Evaporator1/RConn1
  Flow Rate Sensor (2P)1/RConn1 -- Outlet/RConn1
  Flow Rate Sensor (2P)1/RConn2 -- PS-Simulink Converter21/LConn1
  Inlet/RConn1 -- Evaporator1/LConn1
  Flow Rate Sensor (2P)1/LConn1 -- Evaporator1/LConn2

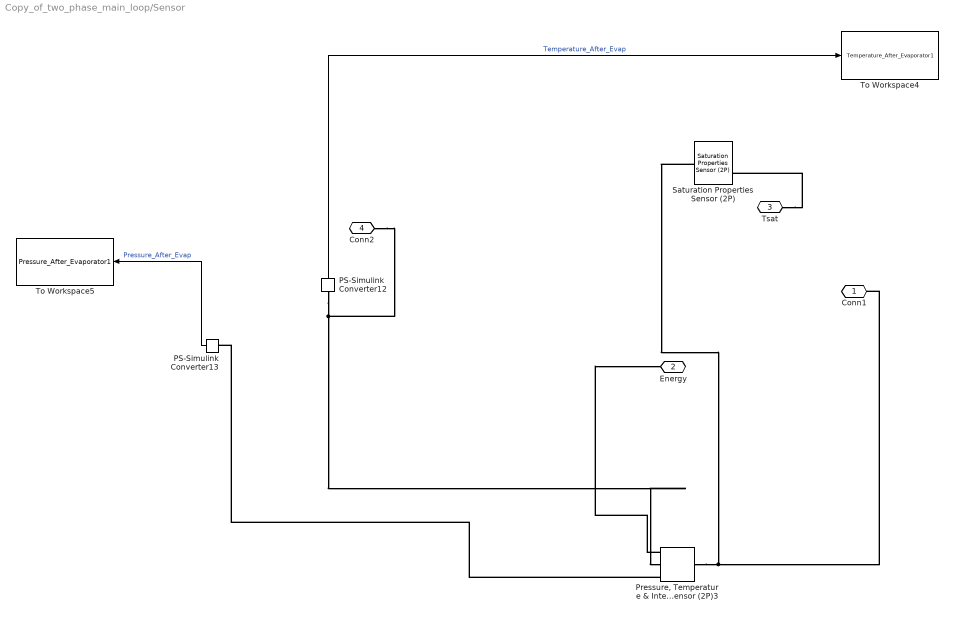
== system Copy_of_two_phase_main_loop/Sensor ==
  PS-Simulink Converter12 : nesl_utility/PS-Simulink Converter  PhysicalDomain=network_engine_domain  SubClassName=ps_output  LeftPortType=input  RightPortType=output  PseudoPeriodic=off  Frequencies=[]  VectorFormat=inherit  Unit=inherit  AffineConversion=off
  PS-Simulink Converter13 : nesl_utility/PS-Simulink Converter  PhysicalDomain=network_engine_domain  SubClassName=ps_output  LeftPortType=input  RightPortType=output  PseudoPeriodic=off  Frequencies=[]  VectorFormat=inherit  Unit=inherit  AffineConversion=off
  "Pressure, Temperature & Internal Energy Sensor (2P)3" : fl_lib/Two-Phase Fluid/Sensors/Pressure, Temperature & Internal Energy Sensor (2P)  reference=foundation.enum.MeasurementReference.absolute  pressure=true  pressure_spec=foundation.enum.PressureMeasementSpec.Absolute  temperature=true  internal_energy=true
      settings: InternalSimscapePortConfiguration="{\"Bottom\":[{\"id\":\"T\",\"label\":\"T\",\"type\":\"output\"},{\"id\":\"U\",\"label\":\"U\",\"type\":\"output\"}],\"Left\":[{\"id\":\"A\",\"label\":\"A\",\"type\":\"foundation.two_phase_fluid.two_phase_fluid\"}],\"Right\":[{\"id\":\"Pa\",\"label\":\"Pa\",\"type\":\"output\"}],\"Top\":[]}"
  Saturation Properties Sensor (2P) : fl_lib/Two-Phase Fluid/Sensors/Saturation Properties Sensor (2P)  temperature_measure=true  pressure_measure=false  pressure_check=simscape.enum.assert.action.error  energy_measure=foundation.enum.EnergyMeasurement.Off  density_measure=foundation.enum.DensityMeasurement.Off
      settings: InternalSimscapePortConfiguration="{\"Bottom\":[],\"Left\":[{\"id\":\"A\",\"label\":\"A\",\"type\":\"foundation.two_phase_fluid.two_phase_fluid\"}],\"Right\":[{\"id\":\"T_sat_liq\",\"label\":\"TL\",\"type\":\"output\"},{\"id\":\"T_sat_vap\",\"label\":\"TV\",\"type\":\"output\"}],\"Top\":[]}"
  To Workspace4 : ToWorkspace  VariableName=Temperature_After_Evaporator1  SampleTime=-1
  To Workspace5 : ToWorkspace  VariableName=Pressure_After_Evaporator1  SampleTime=-1
  Conn1 : PMIOPort  Side=Left
  Energy : PMIOPort  Port=2  Side=Right
  Tsat : PMIOPort  Port=3  Side=Left
  Conn2 : PMIOPort  Port=4  Side=Left
  wires:
  PS-Simulink Converter13/1 -> To Workspace5/1  "Pressure_After_Evap"
  PS-Simulink Converter12/1 -> To Workspace4/1  "Temperature_After_Evap"
  connections:
  "Pressure, Temperature & Internal Energy Sensor (2P)3"/LConn1 -- Saturation Properties Sensor (2P)/LConn1 -- Conn1/RConn1
  "Pressure, Temperature & Internal Energy Sensor (2P)3"/RConn3 -- Energy/RConn1
  "Pressure, Temperature & Internal Energy Sensor (2P)3"/RConn1 -- PS-Simulink Converter13/LConn1
  PS-Simulink Converter12/LConn1 -- Conn2/RConn1 -- "Pressure, Temperature & Internal Energy Sensor (2P)3"/RConn2
  Tsat/RConn1 -- Saturation Properties Sensor (2P)/RConn2

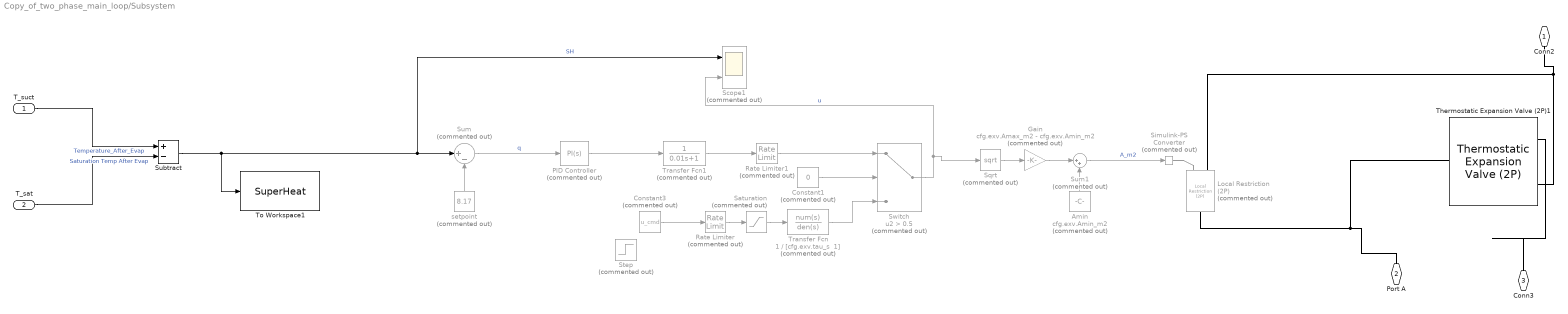
== system Copy_of_two_phase_main_loop/Subsystem ==
  T_suct : Inport
  T_sat : Inport  Port=2
  Amin : Constant  Commented=on  Value=cfg.exv.Amin_m2
  Constant1 : Constant  Commented=on  Value=0
  Constant3 : Constant  Commented=on  Value=u_cmd
  Gain : Gain  Commented=on  Gain=cfg.exv.Amax_m2 - cfg.exv.Amin_m2
  Local Restriction (2P) : fl_lib/Two-Phase Fluid/Elements/Local Restriction (2P)  Commented=on  restriction_type=foundation.enum.restriction_type.variable  restriction_area=1e-3 m^2  min_area="cfg.exv.Amin_m2  m^2"  max_area="cfg.exv.Amax_m2  m^2"  pressure_loss_model=foundation.enum.RestrictionPressureLossModel.Bernoulli  area=pi*0.02^2/4 m^2  Cd=0.64  B_lam=0.999
      settings: InternalSimscapePortConfiguration="{\"Bottom\":[],\"Left\":[{\"id\":\"A\",\"label\":\"A\",\"type\":\"foundation.two_phase_fluid.two_phase_fluid\"},{\"id\":\"area_in\",\"label\":\"AR\",\"type\":\"input\"}],\"Right\":[{\"id\":\"B\",\"label\":\"B\",\"type\":\"foundation.two_phase_fluid.two_phase_fluid\"}],\"Top\":[]}"
  PID Controller : slpidlib/PID Controller  Commented=on  Controller=PI  Form=Parallel  TimeDomain=Continuous-time  UseExternalTs=off  SampleTime=-1  IntegratorMethod=Forward Euler  FilterMethod=Forward Euler  ControllerParametersSource=internal  P=0.05  I=0.0002  UseKiTs=off  D=0  UseExternalDerivativeSource=off  N=100  UseFilter=on  TunerSelectOption=Transfer Function Based (PID Tuner App)  InitialConditionSource=internal  InitialConditionForIntegrator=0  InitialConditionForFilter=0  DifferentiatorICPrevScaledInput=0  ExternalReset=none  TrackingMode=off  Kt=1  LimitOutput=on  SatLimitsSource=internal  UpperSaturationLimit=1  LowerSaturationLimit=0  LinearizeAsGain=on  AntiWindupMode=clamping  Kb=1  LimitIntegrator=on  UpperIntegratorSaturationLimit=1  LowerIntegratorSaturationLimit=0  POutMin=[]  POutMax=[]  IOutMin=[]  IOutMax=[]  DOutMin=[]  DOutMax=[]  NOutMin=[]  NOutMax=[]  SumOutMin=[]  SumOutMax=[]  SaturationOutMin=[]  SaturationOutMax=[]  PParamMin=[]  PParamMax=[]  IParamMin=[]  IParamMax=[]  DParamMin=[]  DParamMax=[]  NParamMin=[]  NParamMax=[]  KbParamMin=[]  KbParamMax=[]  KtParamMin=[]  KtParamMax=[]  KbOutMin=[]  KbOutMax=[]  KtOutMin=[]  KtOutMax=[]  IntegratorOutMin=[]  IntegratorOutMax=[]  FilterOutMin=[]  FilterOutMax=[]  SumI1OutMin=[]  SumI1OutMax=[]  SumI2OutMin=[]  SumI2OutMax=[]  SumI3OutMin=[]  SumI3OutMax=[]  SumI4OutMin=[]  SumI4OutMax=[]  SumDOutMin=[]  SumDOutMax=[]  DifferentiatorOutMin=[]  DifferentiatorOutMax=[]  FilterDiffOutCoefMin=[]  FilterDiffOutCoefMax=[]  ReciprocalOutMin=[]  ReciprocalOutMax=[]  SumDenOutMin=[]  SumDenOutMax=[]  SumNumOutMin=[]  SumNumOutMax=[]  DivideOutMin=[]  DivideOutMax=[]  UdiffTsProdOutMin=[]  UdiffTsProdOutMax=[]  NTsProdOutMin=[]  NTsProdOutMax=[]  UintegralTsProdOutMin=[]  UintegralTsProdOutMax=[]  UngainTsProdOutMin=[]  UngainTsProdOutMax=[]  ClampingZeroOutDataTypeStr=Inherit: Inherit via back propagation  ClampingZeroOutMin=[]  ClampingZeroOutMax=[]  FilterDenConstantOutDataTypeStr=Inherit: Inherit via back propagation  FilterDenConstantOutMin=[]  FilterDenConstantOutMax=[]  PCopyOutDataTypeStr=Inherit: Inherit via back propagation  PCopyOutMin=[]  PCopyOutMax=[]  NCopyOutDataTypeStr=Inherit: Inherit via back propagation  NCopyOutMin=[]  NCopyOutMax=[]  IntegratorContinuousStateAttributes=''  IntegratorStateMustResolveToSignalObject=off  IntegratorRTWStateStorageClass=Auto  FilterContinuousStateAttributes=''  FilterStateMustResolveToSignalObject=off  FilterRTWStateStorageClass=Auto  ParallelPVariant=InternalParameters  IdealPVariant=Disabled  IVariant=InternalParameters  DVariant=Disabled  IntegratorVariant=Continuous  SatVariant=Enabled  AWVariant=ContClampingParallel  PCopyVariant=Disabled  TRVariant=Disabled  FdbkBlocksVariant=Forward  IdealPFdbkVariant=Disabled  SatFdbkVariant=Disabled  DerivativeFilterVariant=Disabled  NVariant=Disabled  NCopyVariant=Disabled_SignalSpec  FilterICVariant=Disabled  IntegratorICVariant=InternalICs  ExternalResetVariant=Disabled  TRSumVariant=Passthrough  SumFdbkVariant=Disabled  SumVariant=Sum_PI  TsampFilterVariant=InternalTs  TsampNgainVariant=Passthrough  TsampIntegralVariant=Disabled_SignalSpec  ExternalSaturationOutDataTypeStr=Inherit: Same as second input  DerivativeSourceVariant=Disabled  PreIntVariant=InternalPreInt
  Rate Limiter : RateLimiter  Commented=on  RisingSlewLimit=0.01  FallingSlewLimit=-0.01  SampleTimeMode=inherited  LinearizeAsGain=off
  Rate Limiter1 : RateLimiter  Commented=on  RisingSlewLimit=100  FallingSlewLimit=- 100  SampleTimeMode=inherited  LinearizeAsGain=off
  Saturation : Saturate  Commented=on  UpperLimit=cfg.exv.u_max  LowerLimit=0
  Scope1 : Scope  Commented=on  NumInputPorts=2
      settings: ActiveDisplayYMinimum=-231.24035158922058  ActiveDisplayYMaximum=311.50161349127353  DataLoggingVariableName=ScopeData3
  Simulink-PS Converter : nesl_utility/Simulink-PS Converter  Commented=on  PhysicalDomain=network_engine_domain  SubClassName=ps_input  LeftPortType=input  RightPortType=output  PseudoPeriodic=off  Frequencies=[]  NoiseDistribution=none  NoiseParameters=[]  Unit=m^2  AffineConversion=off  FilteringAndDerivatives=provide  SimscapeFilterOrder=1  InputFilterTimeConstant=0.001  UdotUserProvided=0
  Sqrt : Sqrt  Commented=on
  Step : Step  Commented=on  Time=200  After=0.2  SampleTime=0
  Subtract : Sum  Inputs=+-
  Sum : Sum  Commented=on  Inputs=|+-
  Sum1 : Sum  Commented=on  Inputs=|++
  Switch : Switch  Commented=on  Criteria=u2 > Threshold  Threshold=0.5  SaturateOnIntegerOverflow=off  InputSameDT=off
  Thermostatic Expansion Valve (2P)1 : SimscapeFluids_lib/Two-Phase Fluid/Valves & Orifices/Flow Control Valves/Thermostatic Expansion Valve (2P)  valve_parameterization=fluids.two_phase_fluid.valves_orifices.flow_control_valves.enum.ThermostaticExpansionValveParameterization.Nominal  capacity_spec=fluids.two_phase_fluid.valves_orifices.flow_control_valves.enum.ThermostaticExpansionValveCapacitySpec.HeatTransfer  Q_nominal=14 kW  Q_max=30 kW  mdot_nominal=0.005 kg/s  mdot_max=0.008 kg/s  pressure_spec=fluids.two_phase_fluid.valves_orifices.flow_control_valves.enum.ThermostaticExpansionValvePressureSpec.SaturationTemperature  p_cond_nominal=1.5 MPa  p_evap_nominal=0.5 MPa  T_cond_nominal=45 degC  T_evap_nominal=5 degC  delta_T_sub=5 deltaK  delta_T_nominal=5 deltaK  delta_T_static=2 deltaK  mop=fluids.two_phase_fluid.valves_orifices.flow_control_valves.enum.ThermostaticExpansionValveMOP.Off  p_mop=0.5 MPa  T_mop=288.15 K  T_evap_out_TLU1=0 : 10 : 40 degC  p_bulb_TLU1=0.3 : 0.1 : 0.7 MPa  lift_TLU2=0 : 0.15 : 0.6 mm  p_evap_TLU2=0.3 : -0.05 : 0.1 MPa  lift_TLU3=0 : 0.15 : 0.6 mm  mdot_TLU3=0 : 0.015 : 0.06 kg/s  p_cond_ref=2 MPa  p_evap_ref=0.2 MPa  T_evap_out_ref=0 degC  delta_T_sub_ref=5 deltaK  pressure_equalization=fluids.two_phase_fluid.valves_orifices.flow_control_valves.enum.ThermostaticExpansionValveEqualization.Internal  bulb_dynamics=false  tau_bulb=20 s  leakage_fraction=1e-6  smoothing_factor=0.01  B_lam=0.999  tau_x=0.1 s  area=pi*0.02^2/4 m^2
      settings: InternalSimscapePortConfiguration="{\"Bottom\":[],\"Left\":[{\"id\":\"A\",\"label\":\"A\",\"type\":\"foundation.two_phase_fluid.two_phase_fluid\"}],\"Right\":[{\"id\":\"B\",\"label\":\"B\",\"type\":\"foundation.two_phase_fluid.two_phase_fluid\"}],\"Top\":[{\"id\":\"S\",\"label\":\"S\",\"type\":\"foundation.two_phase_fluid.two_phase_fluid\"}]}"
  To Workspace1 : ToWorkspace  VariableName=SuperHeat  SampleTime=-1
  Transfer Fcn : TransferFcn  Commented=on  Numerator=1  Denominator="[cfg.exv.tau_s  1]"
  Transfer Fcn1 : TransferFcn  Commented=on  Numerator=1  Denominator="[0.01  1]"
  setpoint : Constant  Commented=on  Value=8.17
  Conn2 : PMIOPort  Side=Left
  Port A : PMIOPort  Port=2  Side=Right
  Conn3 : PMIOPort  Port=3  Side=Right
  wires:
  Switch/1 -> Scope1/2, Sqrt/1  "u"
  Transfer Fcn1/1 -> Rate Limiter1/1
  Constant1/1 -> Switch/2
  Rate Limiter/1 -> Saturation/1
  Transfer Fcn/1 -> Switch/3
  Subtract/1 -> To Workspace1/1, Scope1/1, Sum/1  "SH"
  Sum1/1 -> Simulink-PS Converter/1  "A_m2"
  T_suct/1 -> Subtract/1  "Temperature_After_Evap"
  T_sat/1 -> Subtract/2  "Saturation Temp After Evap"
  Sqrt/1 -> Gain/1
  Gain/1 -> Sum1/1
  Amin/1 -> Sum1/2
  setpoint/1 -> Sum/2
  Rate Limiter1/1 -> Switch/1
  Saturation/1 -> Transfer Fcn/1
  Sum/1 -> PID Controller/1  "q"
  PID Controller/1 -> Transfer Fcn1/1
  Constant3/1 -> Rate Limiter/1
  connections:
  Simulink-PS Converter/RConn1 -- Local Restriction (2P)/LConn2
  Conn3/RConn1 -- Thermostatic Expansion Valve (2P)1/LConn2
  Conn2/RConn1 -- Thermostatic Expansion Valve (2P)1/LConn1 -- Local Restriction (2P)/LConn1
  Port A/RConn1 -- Thermostatic Expansion Valve (2P)1/RConn1 -- Local Restriction (2P)/RConn1

== matlab function Copy_of_two_phase_main_loop/Calculation: mdot˙(hout​−hin​)/MATLAB Function ==
  data: h_in_kJpkg input; ton output; h_out_kJpkg input; mdot_kgps input
function ton = calc_tonnage(h_in_kJpkg, h_out_kJpkg, mdot_kgps)
%   calc_tonnage  Computes system capacity in refrigeration tons.
%
%   ton = calc_tonnage(h_in_kJpkg, h_out_kJpkg, mdot_kgps, mode)
%
%   Inputs
%   -------
%   h_in_kJpkg   : inlet specific enthalpy  [kJ/kg]
%   h_out_kJpkg  : outlet specific enthalpy [kJ/kg]
%   mdot_kgps    : mass flow rate           [kg/s]
%
%   Output
%   -------
%   ton          : capacity in refrigeration tons [TR]
%
%   Notes
%   -----
%   • For evaporators (cooling): Q̇ = ṁ × (h_out − h_in)
%   • 1 ton refrigeration = 3.517 kW
%
%   Example
%   -------
%       ton_cool = calc_tonnage(250, 430, 0.05);
%


Qdot_kW = mdot_kgps .* (h_out_kJpkg - h_in_kJpkg); % kJ/kg × kg/s = kJ/s = kW


ton = Qdot_kW ./ 3.517; % Convert to refrigeration tons

end
